simulink model "prototipo"  (R2022b)
settings: Solver=ode3  StartTime=0.0  StopTime=10  RelTol=1e-3  EnableMultiTasking=on
model workspace (MAT data in the model file):
  RGBData = [62 63 65 64 60 62 65 62 60 59 59 59 ... (230400 elements, 320x240x3)]
libraries: sensehatlib x2, raspberrypiAVlib x2, visionanalysis x1, visiontextngfix x1
(part 2 of 2)

== matlab function prototipo/MATLAB Function ==
  data: image input; output output; label input

function output = addLabel(image,label)
%#codegen
label_str = cellstr(label);
text2display = sprintf("Label : %s \nScore: %f", label_str{:}, max_score);
% Para la generación de código, text2display necesita ser de tipo cell
% en vez de string
ctext2display = cellstr(text2display);
% Insertamos en img, en la posición 0,0, el texto previamente calculado
output = insertText(image, [0,0], ctext2display);
end

== matlab function prototipo/MATLAB Function1 ==
  data: i input; r output; g output; b output
function [r,g,b] = ImageToRGB(i)
%#codegen
r =i(:,:,1);
g =i(:,:,2);
b =i(:,:,3);
end
